simulink model "Alireza_Abassi1"  (R2021a)
settings: Solver=VariableStepAuto  StartTime=0.0  StopTime=3  RelTol=1e-3
values from neighbouring files (symbols this model uses):
  A = [0,  1,  0,  0,  0,  0 ... (first row only)    [Taklif.m]
  A1 = [0,     1,      0,       0 ... (first row only)    [Taklif.m]
  A2 = [0,    1 ... (first row only)    [Taklif.m]
  B = [0,     0 ... (first row only)    [Taklif.m]
  B1 = [0;  0.3803;   0;    -2.3629]    [Taklif.m]
  B2 = [0;   0.5085]    [Taklif.m]
  C = [0, 1,  0,  0,  0,  0 ... (first row only)    [Taklif.m]
  C1 = [0 1 0 0 ... (first row only)    [Taklif.m]
  C2 = [0 1]    [Taklif.m]
  K1 = place(A, B, [-2 -3 -4 -5 -4.5 -3.2])    [Taklif.m]
  K2 = lqr(A2, B2, Q2, R2)    [Taklif.m]
undefined symbols (not defined in the file or in its folder): K
settings Model: Creator=alire  LastModifiedBy=alire

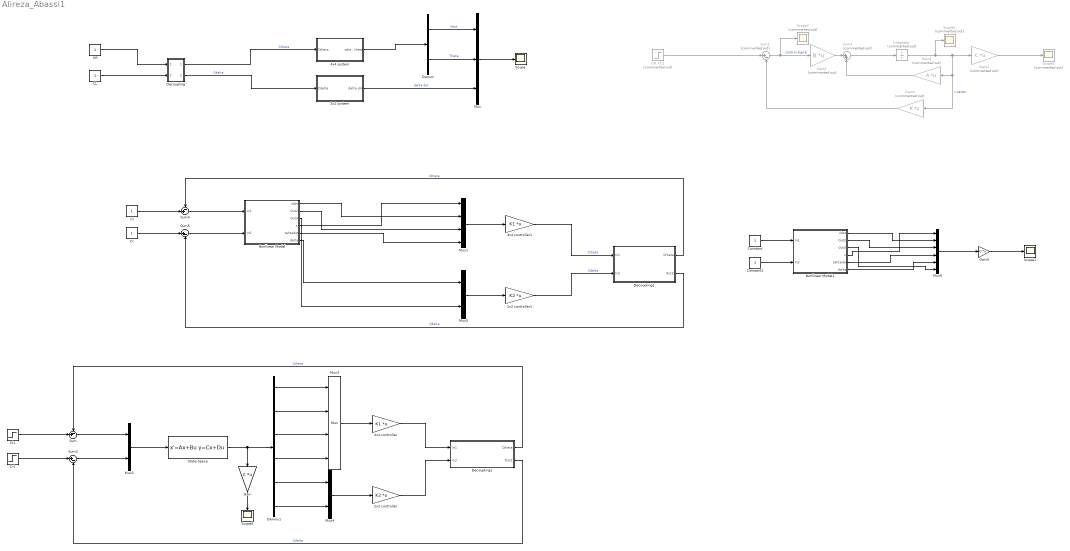
== system Alireza_Abassi1 ==
  2x2 controller : Gain  Gain=K2  Multiplication=Matrix(K*u)
  2x2 controller1 : Gain  Gain=K2  Multiplication=Matrix(K*u)
  2x2 system : Subsystem
  4x4 controller : Gain  Gain=K1  Multiplication=Matrix(K*u)
  4x4 controller1 : Gain  Gain=K1  Multiplication=Matrix(K*u)
  4x4 system : Subsystem
  CL : Constant
  CR : Constant
  "CR, CL1" : Step  Commented=on  Before=[0; 0]  After=[1; 1]  SampleTime=0
  Cl : Constant
  Cl1 : Step  Time=0.01  Before=1  After=0  SampleTime=0
  Constant : Constant
  Constant1 : Constant
  Cr : Constant
  Cr1 : Step  Time=0.01  Before=1  After=0  SampleTime=0
  Decoupling : Subsystem
  Decoupling1 : Subsystem
  Decoupling2 : Subsystem
  Demux : Demux  Outputs=2
  Demux1 : Demux  Outputs=6
  Gain : Gain  Gain=C  Multiplication=Matrix(K*u)
  Gain1 : Gain  Commented=on  Gain=B  Multiplication=Matrix(K*u) (u vector)
  Gain2 : Gain  Commented=on  Gain=C  Multiplication=Matrix(K*u) (u vector)
  Gain3 : Gain  Commented=on  Gain=A  Multiplication=Matrix(K*u) (u vector)
  Gain4 : Gain  Commented=on  Gain=K  Multiplication=Matrix(K*u) (u vector)
  Gain5 : Gain  Gain=C  Multiplication=Matrix(K*u)
  Integrator : Integrator  Commented=on
  Mux : Mux  Inputs=3
  Mux1 : Mux
  Mux2 : Mux  Inputs=2
  Mux3 : Mux
  Mux4 : Mux  Inputs=2
  Mux5 : Mux  Inputs=2
  Mux6 : Mux  Inputs=6
  Nonlinear Model : Subsystem
  Nonlinear Model1 : Subsystem
  Scope : Scope
  Scope1 : Scope
  Scope2 : Scope  Commented=on
  Scope3 : Scope  Commented=on
  Scope4 : Scope  Commented=on
  Scope5 : Scope
  State-Space : StateSpace  A=A  B=B  C=eye(6)  D=zeros(6, 2)  InitialCondition=0
  Sum : Sum  Inputs=-+|
  Sum1 : Sum  Commented=on  Inputs=|+-
  Sum2 : Sum  Commented=on  Inputs=|++
  Sum3 : Sum  Inputs=|+-
  Sum4 : Sum  Inputs=-+|
  Sum5 : Sum  Inputs=|+-
  wires:
  Mux/1 -> Scope/1
  CR/1 -> Decoupling/1(In1)
  CL/1 -> Decoupling/2(In2)
  Demux/1 -> Mux/1  "Xdot"
  Demux/2 -> Mux/2  "Theta"
  Decoupling/2(Out2) -> 2x2 system/1(Cdelta)  "Cdelta"
  2x2 system/1(delta dot) -> Mux/3  "delta dot"
  Decoupling/1(Ctheta) -> 4x4 system/1(Ctheta)  "Ctheta"
  4x4 system/1("xdot , theta") -> Demux/1
  Gain2/1 -> Scope3/1
  Gain3/1 -> Sum2/2
  Sum1/1 -> Scope4/1, Gain1/1  "control signal"
  Sum2/1 -> Integrator/1
  "CR, CL1"/1 -> Sum1/1
  Integrator/1 -> Gain2/1, Gain4/1, Gain3/1, Scope2/1  "x vector"
  Gain1/1 -> Sum2/1
  Gain4/1 -> Sum1/2
  Mux2/1 -> State-Space/1
  State-Space/1 -> Gain/1, Demux1/1
  Demux1/1 -> Mux3/1
  Demux1/2 -> Mux3/2
  Demux1/3 -> Mux3/3
  Demux1/4 -> Mux3/4
  Mux3/1 -> 4x4 controller/1
  Demux1/5 -> Mux4/1
  Demux1/6 -> Mux4/2
  Mux4/1 -> 2x2 controller/1
  4x4 controller/1 -> Decoupling1/1(In1)
  2x2 controller/1 -> Decoupling1/2(In2)
  Cl1/1 -> Sum/2
  Decoupling1/1(Ctheta) -> Sum/1  "Ctheta"
  Cr1/1 -> Sum3/1
  Sum3/1 -> Mux2/2
  Decoupling1/2(Out2) -> Sum3/2  "Cdelta"
  Sum/1 -> Mux2/1
  Gain/1 -> Scope5/1
  Mux5/1 -> 2x2 controller1/1
  Nonlinear Model/3(Out3) -> Mux5/2
  Nonlinear Model/6(delta) -> Mux5/1
  Mux1/1 -> 4x4 controller1/1
  Sum4/1 -> Nonlinear Model/1(In1)
  Sum5/1 -> Nonlinear Model/2(In2)
  Nonlinear Model/4(x) -> Mux1/1
  Nonlinear Model/1(xdot) -> Mux1/2
  Nonlinear Model/2(Out2) -> Mux1/3
  Nonlinear Model/5(tehtadot) -> Mux1/4
  4x4 controller1/1 -> Decoupling2/1(In1)  "Ctheta"
  2x2 controller1/1 -> Decoupling2/2(In2)  "Cdelta"
  Cl/1 -> Sum4/2
  Cr/1 -> Sum5/1
  Decoupling2/1(Ctheta) -> Sum4/1  "Ctheta"
  Decoupling2/2(Out2) -> Sum5/2  "Cdelta"
  Nonlinear Model1/6(delta) -> Mux6/5
  Nonlinear Model1/5(tehtadot) -> Mux6/4
  Nonlinear Model1/4(x) -> Mux6/1
  Nonlinear Model1/3(Out3) -> Mux6/6
  Nonlinear Model1/2(Out2) -> Mux6/3
  Nonlinear Model1/1(xdot) -> Mux6/2
  Mux6/1 -> Gain5/1
  Gain5/1 -> Scope1/1
  Constant/1 -> Nonlinear Model1/1(In1)
  Constant1/1 -> Nonlinear Model1/2(In2)

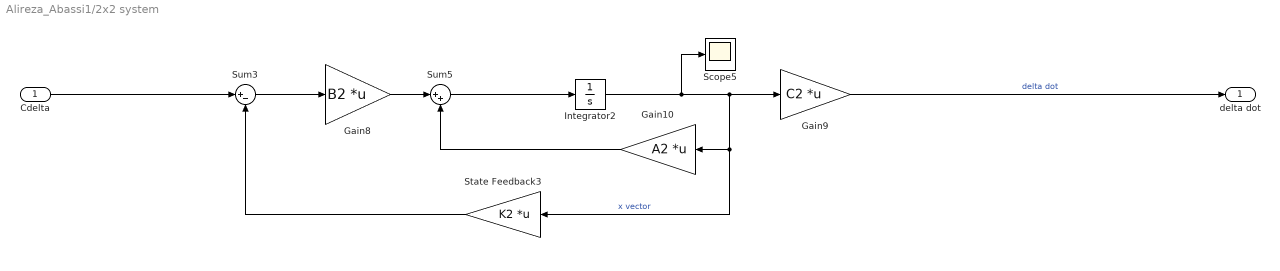
== system Alireza_Abassi1/2x2 system ==
  Cdelta : Inport
  Gain10 : Gain  Gain=A2  Multiplication=Matrix(K*u)
  Gain8 : Gain  Gain=B2  Multiplication=Matrix(K*u)
  Gain9 : Gain  Gain=C2  Multiplication=Matrix(K*u)
  Integrator2 : Integrator  InitialCondition=[1; 0]
  Scope5 : Scope
  State Feedback3 : Gain  Gain=K2  Multiplication=Matrix(K*u)
  Sum3 : Sum  Inputs=|+-
  Sum5 : Sum  Inputs=|++
  delta dot : Outport
  wires:
  Integrator2/1 -> Gain9/1, State Feedback3/1, Gain10/1, Scope5/1  "x vector"
  Gain9/1 -> delta dot/1  "delta dot"
  Sum5/1 -> Integrator2/1
  Gain8/1 -> Sum5/1
  Gain10/1 -> Sum5/2
  Sum3/1 -> Gain8/1
  State Feedback3/1 -> Sum3/2
  Cdelta/1 -> Sum3/1

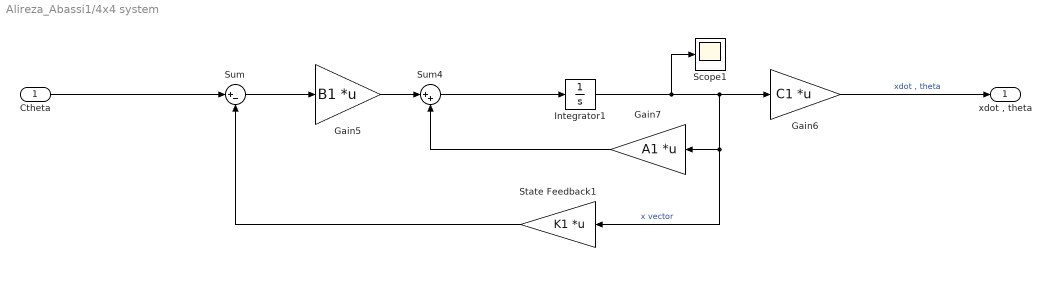
== system Alireza_Abassi1/4x4 system ==
  Ctheta : Inport
  Gain5 : Gain  Gain=B1  Multiplication=Matrix(K*u)
  Gain6 : Gain  Gain=C1  Multiplication=Matrix(K*u)
  Gain7 : Gain  Gain=A1  Multiplication=Matrix(K*u)
  Integrator1 : Integrator  InitialCondition=[1;1;1;1]
  Scope1 : Scope
  State Feedback1 : Gain  Gain=K1  Multiplication=Matrix(K*u)
  Sum : Sum  Inputs=|+-
  Sum4 : Sum  Inputs=|++
  "xdot , theta" : Outport
  wires:
  State Feedback1/1 -> Sum/2
  Integrator1/1 -> Gain6/1, State Feedback1/1, Gain7/1, Scope1/1  "x vector"
  Sum/1 -> Gain5/1
  Sum4/1 -> Integrator1/1
  Gain7/1 -> Sum4/2
  Gain5/1 -> Sum4/1
  Ctheta/1 -> Sum/1
  Gain6/1 -> "xdot , theta"/1  "xdot , theta"

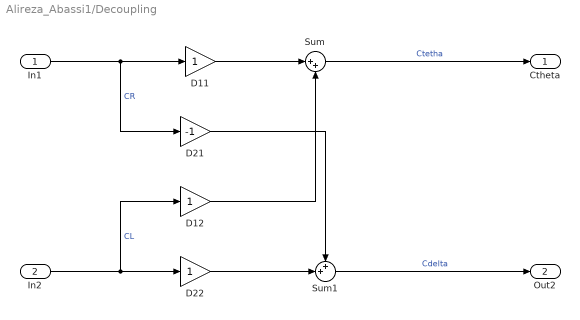
== system Alireza_Abassi1/Decoupling ==
  In1 : Inport
  In2 : Inport  Port=2
  D11 : Gain
  D12 : Gain
  D21 : Gain  Gain=-1
  D22 : Gain
  Sum : Sum  Inputs=|++
  Sum1 : Sum  Inputs=++|
  Ctheta : Outport
  Out2 : Outport  Port=2
  wires:
  Sum1/1 -> Out2/1  "Cdelta"
  D12/1 -> Sum/2
  D21/1 -> Sum1/1
  In2/1 -> D22/1, D12/1  "CL"
  D11/1 -> Sum/1
  D22/1 -> Sum1/2
  In1/1 -> D21/1, D11/1  "CR"
  Sum/1 -> Ctheta/1  "Ctetha"

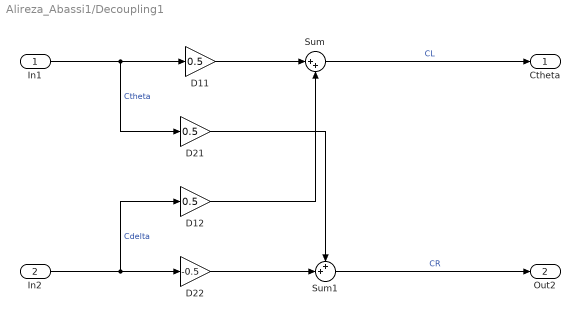
== system Alireza_Abassi1/Decoupling1 ==
  In1 : Inport
  In2 : Inport  Port=2
  D11 : Gain  Gain=0.5
  D12 : Gain  Gain=0.5
  D21 : Gain  Gain=0.5
  D22 : Gain  Gain=-0.5
  Sum : Sum  Inputs=|++
  Sum1 : Sum  Inputs=++|
  Ctheta : Outport
  Out2 : Outport  Port=2
  wires:
  Sum1/1 -> Out2/1  "CR"
  D12/1 -> Sum/2
  D21/1 -> Sum1/1
  In2/1 -> D22/1, D12/1  "Cdelta"
  D11/1 -> Sum/1
  D22/1 -> Sum1/2
  In1/1 -> D21/1, D11/1  "Ctheta"
  Sum/1 -> Ctheta/1  "CL"

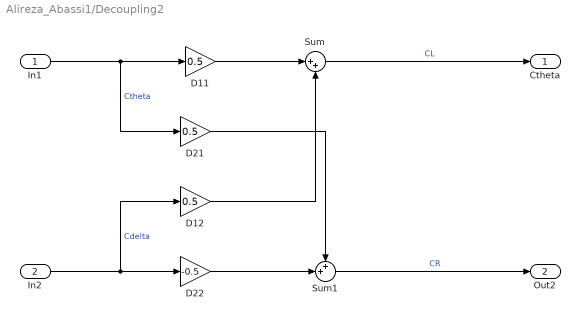
== system Alireza_Abassi1/Decoupling2 ==
  In1 : Inport
  In2 : Inport  Port=2
  D11 : Gain  Gain=0.5
  D12 : Gain  Gain=0.5
  D21 : Gain  Gain=0.5
  D22 : Gain  Gain=-0.5
  Sum : Sum  Inputs=|++
  Sum1 : Sum  Inputs=++|
  Ctheta : Outport
  Out2 : Outport  Port=2
  wires:
  Sum1/1 -> Out2/1  "CR"
  D12/1 -> Sum/2
  D21/1 -> Sum1/1
  In2/1 -> D22/1, D12/1  "Cdelta"
  D11/1 -> Sum/1
  D22/1 -> Sum1/2
  In1/1 -> D21/1, D11/1  "Ctheta"
  Sum/1 -> Ctheta/1  "CL"

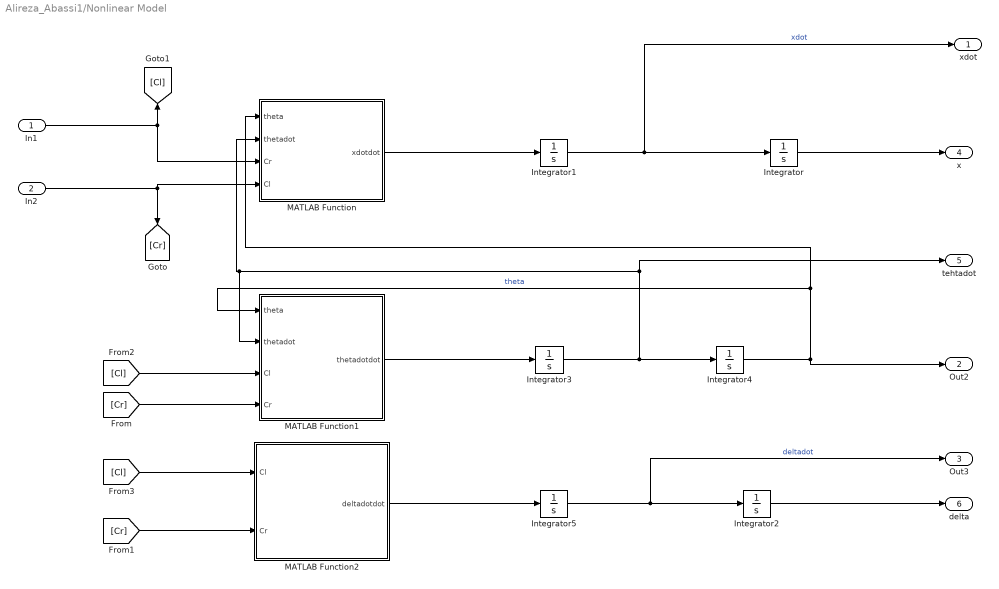
== system Alireza_Abassi1/Nonlinear Model ==
  In1 : Inport
  In2 : Inport  Port=2
  Integrator{,1..5} (6 alike) : Integrator
  MATLAB Function : MATLAB Function  TreatAsAtomicUnit=on
  MATLAB Function1 : MATLAB Function  TreatAsAtomicUnit=on
  MATLAB Function2 : MATLAB Function  TreatAsAtomicUnit=on
  xdot : Outport
  Out2 : Outport  Port=2
  Out3 : Outport  Port=3
  x : Outport  Port=4
  tehtadot : Outport  Port=5
  delta : Outport  Port=6
  wires:
  [Cr] -> MATLAB Function1/4(Cr)
  [Cl] -> MATLAB Function2/1(Cl)
  [Cl] -> MATLAB Function1/3(Cl)
  Integrator1/1 -> xdot/1, Integrator/1  "xdot"
  In1/1 -> MATLAB Function/3(Cr), [Cl]
  Integrator3/1 -> tehtadot/1, MATLAB Function1/2(thetadot), MATLAB Function/2(thetadot), Integrator4/1
  In2/1 -> MATLAB Function/4(Cl), [Cr]
  [Cr] -> MATLAB Function2/2(Cr)
  Integrator5/1 -> Out3/1, Integrator2/1  "deltadot"
  MATLAB Function/1(xdotdot) -> Integrator1/1
  MATLAB Function2/1(deltadotdot) -> Integrator5/1
  MATLAB Function1/1(thetadotdot) -> Integrator3/1
  Integrator4/1 -> MATLAB Function1/1(theta), MATLAB Function/1(theta), Out2/1  "theta"
  Integrator/1 -> x/1
  Integrator2/1 -> delta/1

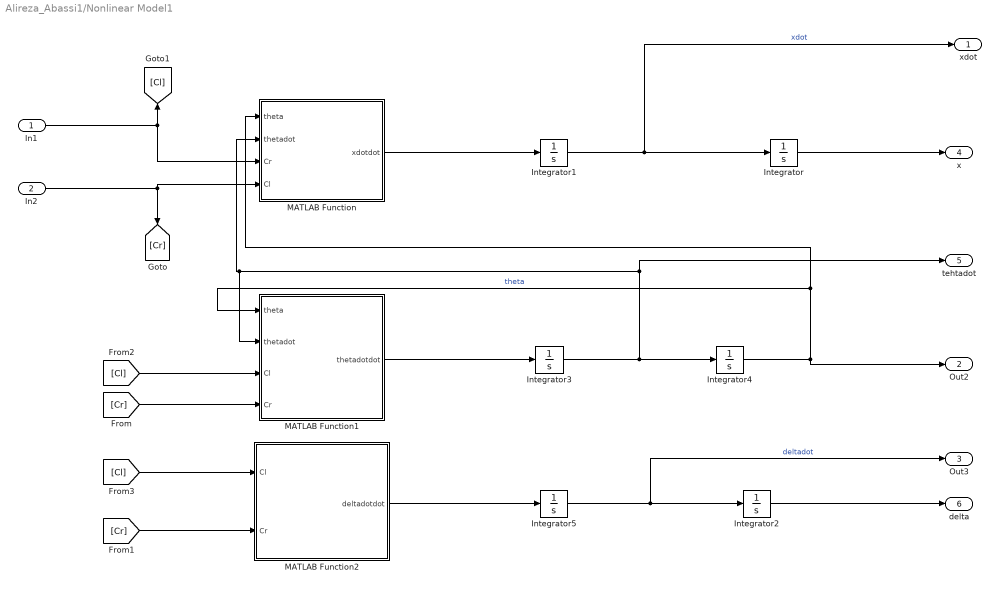
== system Alireza_Abassi1/Nonlinear Model1 ==
  In1 : Inport
  In2 : Inport  Port=2
  Integrator{,1..5} (6 alike) : Integrator
  MATLAB Function : MATLAB Function  TreatAsAtomicUnit=on
  MATLAB Function1 : MATLAB Function  TreatAsAtomicUnit=on
  MATLAB Function2 : MATLAB Function  TreatAsAtomicUnit=on
  xdot : Outport
  Out2 : Outport  Port=2
  Out3 : Outport  Port=3
  x : Outport  Port=4
  tehtadot : Outport  Port=5
  delta : Outport  Port=6
  wires:
  [Cr] -> MATLAB Function1/4(Cr)
  [Cl] -> MATLAB Function2/1(Cl)
  [Cl] -> MATLAB Function1/3(Cl)
  Integrator1/1 -> xdot/1, Integrator/1  "xdot"
  In1/1 -> MATLAB Function/3(Cr), [Cl]
  Integrator3/1 -> tehtadot/1, MATLAB Function1/2(thetadot), MATLAB Function/2(thetadot), Integrator4/1
  In2/1 -> MATLAB Function/4(Cl), [Cr]
  [Cr] -> MATLAB Function2/2(Cr)
  Integrator5/1 -> Out3/1, Integrator2/1  "deltadot"
  MATLAB Function/1(xdotdot) -> Integrator1/1
  MATLAB Function2/1(deltadotdot) -> Integrator5/1
  MATLAB Function1/1(thetadotdot) -> Integrator3/1
  Integrator4/1 -> MATLAB Function1/1(theta), MATLAB Function/1(theta), Out2/1  "theta"
  Integrator/1 -> x/1
  Integrator2/1 -> delta/1

== matlab function Alireza_Abassi1/Nonlinear Model/MATLAB Function1 ==
  data: theta input; thetadot input; thetadotdot output; Cl input; Cr input
function thetadotdot  = fcn(theta,thetadot,Cl,Cr)
mp = 20;
mw = 6;
l = 0.2;
jpy = 1.33;
r = 0.2;
d = 0.5;
jp = 0.27;
jw = 0.12;
g = 9.82;
frr = 0;
frl = 0;
fp = 0;
thetadotdot = -1/(jp*(2*(jw/r^2+mw)+mp)+2*(jw/r^2+mw)*mp*l^2+mp^2*l^2*sin(theta)^2)*(mp^2*l^2*sin(theta)*cos(theta)*thetadot^2+(2*(jw/r^2+mw)+mp)*mp*g*l*sin(theta)-(mp*l*cos(theta)/r+2*(jw/r^2+mw)+mp)*(Cr+Cl)-mp*l*cos(theta)*(frr+frl)+2*(jw/r^2+mw)*l*cos(theta)*fp);

== matlab function Alireza_Abassi1/Nonlinear Model/MATLAB Function ==
  data: theta input; thetadot input; xdotdot output; Cr input; Cl input
function xdotdot = fcn(theta,thetadot,Cr,Cl)

mp = 20;
mw = 6;
l = 0.2;
jpy = 1.33;
r = 0.2;
d = 0.5;
jp = 0.27;
jw = 0.12;
g = 9.82;
frr = 0;
frl = 0;


xdotdot = 1/(jp*(2*(jw/r^2+mw)+mp)+2*(jw/r^2+mw)*mp*l^2+mp^2*l^2*sin(theta)^2)*((jp+mp*l^2)*mp*l*sin(theta)*cos(theta)*thetadot^2-mp^2*l^2*g*cos(theta)*sin(theta)+(1/r*(jp+mp*l^2)+mp*l*cos(theta))*(Cr+Cl)+(jp+mp*l^2*(frr+frl)));

== matlab function Alireza_Abassi1/Nonlinear Model/MATLAB Function2 ==
  data: Cl input; deltadotdot output; Cr input
function deltadotdot = fcn(Cl, Cr)
mp = 20;
mw = 6;
l = 0.2;
jpy = 1.33;
r = 0.2;
d = 0.5;
jp = 0.27;
jw = 0.12;
g = 9.82;
fr = 0;
fl = 0;

deltadotdot = ((Cl-Cr)/r+(fl-fr))/(2*jp*mw+jw*d/r^2);

== matlab function Alireza_Abassi1/Nonlinear Model1/MATLAB Function ==
  data: theta input; thetadot input; xdotdot output; Cr input; Cl input
function xdotdot = fcn(theta,thetadot,Cr,Cl)

mp = 20;
mw = 6;
l = 0.2;
jpy = 1.33;
r = 0.2;
d = 0.5;
jp = 0.27;
jw = 0.12;
g = 9.82;
frr = 0;
frl = 0;


xdotdot = 1/(jp*(2*(jw/r^2+mw)+mp)+2*(jw/r^2+mw)*mp*l^2+mp^2*l^2*sin(theta)^2)*((jp+mp*l^2)*mp*l*sin(theta)*cos(theta)*thetadot^2-mp^2*l^2*g*cos(theta)*sin(theta)+(1/r*(jp+mp*l^2)+mp*l*cos(theta))*(Cr+Cl)+(jp+mp*l^2*(frr+frl)));

== matlab function Alireza_Abassi1/Nonlinear Model1/MATLAB Function1 ==
  data: theta input; thetadot input; thetadotdot output; Cl input; Cr input
function thetadotdot  = fcn(theta,thetadot,Cl,Cr)
mp = 20;
mw = 6;
l = 0.2;
jpy = 1.33;
r = 0.2;
d = 0.5;
jp = 0.27;
jw = 0.12;
g = 9.82;
frr = 0;
frl = 0;
fp = 0;
thetadotdot = -1/(jp*(2*(jw/r^2+mw)+mp)+2*(jw/r^2+mw)*mp*l^2+mp^2*l^2*sin(theta)^2)*(mp^2*l^2*sin(theta)*cos(theta)*thetadot^2+(2*(jw/r^2+mw)+mp)*mp*g*l*sin(theta)-(mp*l*cos(theta)/r+2*(jw/r^2+mw)+mp)*(Cr+Cl)-mp*l*cos(theta)*(frr+frl)+2*(jw/r^2+mw)*l*cos(theta)*fp);

== matlab function Alireza_Abassi1/Nonlinear Model1/MATLAB Function2 ==
  data: Cl input; deltadotdot output; Cr input
function deltadotdot = fcn(Cl, Cr)
mp = 20;
mw = 6;
l = 0.2;
jpy = 1.33;
r = 0.2;
d = 0.5;
jp = 0.27;
jw = 0.12;
g = 9.82;
fr = 0;
fl = 0;

deltadotdot = ((Cl-Cr)/r+(fl-fr))/(2*jp*mw+jw*d/r^2);
